simulink library "simetranss"  (R2024b)
settings: Solver=VariableStepAuto  StartTime=0.0  StopTime=10.0  RelTol=1e-3
PostLoadFcn:
  | Ts=1e-6
InitFcn:
  | Ts=1e-6
undefined symbols (not defined in the file): C, C_601, C_603, C_606, CC, Csnu, Csnubber, DiscIntNeverNeededParam, DPL, DPL1ph, FluxTable, ft2km, gcbh, h, Half, Imap2, L, L_601, L_603, L_606, Lbase, LpejoSw, Newton, R_601, R_603, R_606, Raphson, ResistanceM, Roff, Ron, RotorAngles, Rsnu, Rsnubber, Rt4, SampleTime, simetran, sps, sps_rtmsupport, StatorCurrents, T_2wind_ratio, T_Lpu, T_Lpu_pri, T_Rpu, T_Rpu_pri, T_Vpri, T_Vpri_15comp, T_Vsec, Ti, Ts_Power, Z, Zbase, Zm
libraries: fl_lib x248, ee_lib x146, nesl_utility x122, $bdroot x29, simulink x15, eeGeneralControl x2, spsStairGeneratorLib x2, artemis x1
(part 2 of 12)

== system simetranss/Machines ==
  note: Alternative PMSM/BLDC models
  MATE 6/4 SRM : Subsystem  mask(MATE 6/4 Switched Reluctance Motor){MachineType=6/4, Rs=0.05, Inertia=0.05, FluxTable=FluxTable, RotorAngles=RotorAngles, StatorCurrents=StatorCurrents, Friction=0.02, Initialangle=0, TsBlock=-1, nb_points=[100,20,20], PlotCurves=on}
      mask prompts: MachineType "Type:"; Rs "Stator resistance (Ohms):"; Inertia "Inertia (kg.m.m):"; FluxTable "Magnetization characteristic table:"; RotorAngles "Rotor angle vector (degrees):"; StatorCurrents "Stator current vector (A):"; Friction "Friction (N.m.s):"; Initialangle "Initial position (Deg):"; TsBlock "Sample time (-1 for inherited):"; nb_points "Tables Resampling: [flux, angles, currents]"; PlotCurves "Plot magnetization curves"
      mask help:
      | Models a 6/4 switch reluctance motor in MATE-SimScape.
      |
      | See MATE_SwitchedReluctanceMotor64Drive.slx for detailed explanations.
      mask init:
      | block = gcb ;
      | 
      | 
      | %icon
      | x=[-40 -38 -36 -35:5:35  36 38 40];
      | y=round(sqrt(40*40-x.*x));
      | ym=-y;
      | x1=[-35 -33 -31 -30:5:30 31 33 35]/5;
      | y1=round(sqrt(35*35/25-x1.*x1));
      | ym1=-y1;
      | 
      | typ=get_param(block,'MachineType');
      | 
      | table_mode=1;
      | fluxmatfile=FluxTable;
      | srmtype='6/4';
      | theta=RotorAngles;
      | Icoil=StatorCurrents ;
      | currentmap=1;curthetaaxis=1;curfluxaxis=1;torquemap=1;tethetaaxis=1;tecuraxis=1;
      | plotdata=get_param(block,'PlotCurves');
      | init_rotor_pos=[0 -30 -60]+Initialangle;
      | 
      | 
      | [Icoil2,theta2,Imap2, Temap, all_flux_value]=MATE_SRMparam(table_mode,...
      |     fluxmatfile,theta,Icoil,...
      |     currentmap,curthetaaxis,curfluxaxis,...
      |     torquemap,tethetaaxis,tecuraxis,...
      |     srmtype,plotdata,nb_points);
      mask TypeOptions MachineType: 6/4
      mask DialogControl Container2 Prompt: Parameters
  MATE Brushless DC Motor (ALT1) : Subsystem  mask(Round-Rotor PMSM  (Fixed Admittance)){Rs=0.12, Ld=0.003, Mf=0.25366, pp=3, AngInit=0, Ts=Ts}
      mask prompts: Rs "Stator resistance (Ohms)"; Ld "Stator inductance (H)"; Mf "Magnet flux (Wb)"; pp "Number of pairs of poles"; AngInit "Initial mechanical angle (deg)"; Ts "Sample Time (s)"
      mask help:
      | Implements a three-phase round-rotor permanent magnet synchronous machine with stator windings connected in wye to an internal neutral point.
      |
      | Magnet flux is aligned with the d-axis and therefore a sinusoidal back EMF waveform is assumed by the model.
      |
      | The round rotor assumption is equivalent to Ld=Lq. The phase domain inductance matrix is constant in time.
      |
      | This PMSM model is designed with a fixed admittance from the point of view of the SimScape solver and therefore excellent for real-time simulation and HDL coder.
      |
      |
      | Simulink input: Mechanical rotor speed (rad/s)
      |
      | Parameters:
      | Stator resistance in Ohms
      | Stator inductance in Henry (assume Ld=Lq)
      | Magnet flux in Weber: this is the peak magnet flux seen by the stator windings.
      | Number of pairs of poles.
      | Initial angle of the rotor in degrees.
      | Sample time in seconds
  MATE Induction Machine : Subsystem  mask(MATE Induction Machine){Rs=0.5968, Lls=0.0003495, Rr=0.6258, Llr=0.005473, Lm=0.0354, pp=2, Ts=Ts, disc=Backward Euler, park=Stationary, Parameter11=}
      mask prompts: Rs "Stator resistance (Ohms)"; Lls "Stator leakeage inductance (H)"; Rr "Rotor resistance (seen from stator) (Ohms)"; Llr "Rotor leakeage inductance (seen from stator) (H)"; Lm "Mutual inductance (H)"; pp "Number of pairs of poles"; Ts "Sample Time (s)"; disc "Discretization"; park "D-Q reference frame"
      mask help:
      | The MATE induction machine implements a three-phase asynchronous machine (squirrel cage) modeled with a fixed or rotot-based dq reference frame. Stator and rotor windings are connected in wye to an internal neutral point.
      |
      | This model provides a constant admittance to the DAE SimScape solver and make it directly usable in HDL Coder.
      |
      | In particular, there is no matrix inversion occuring in the model when selecting the Stationary frame of reference.
      |
      | Inputs: w_mec: the mechanical frequency of the rotor in rad/s.
      mask init:
      | dis=get_param(gcb,'disc');
      | if isequal(dis,'Backward Euler')
      |     be='on';
      |     ben=1;
      | else
      |     be='off';
      |     ben=0;
      | end
      | 
      | parkk=get_param(gcb,'park');
      | 
      | if isequal(parkk,'Stationary')
      |     park_num=1;
      | else
      |     park_num=0;
      | end
      | 
      | 
      | Lr=Lm+Llr;
      | Ls=Lm+Lls;
      | 
      | invLmat=1/(Lr*Ls-Lm*Lm)*[Lr 0 -Lm 0; 0 Lr 0 -Lm; -Lm 0  Ls  0;  0  -Lm  0  Ls];
      | moinsRmat=-[Rs 0 0 0; 0 Rs 0 0; 0 0  Rr  0;  0  0  0  Rr];
      | Ac=moinsRmat*invLmat;
      | 
      | 
      | 
      | T=[1 0;0 1]*sqrt(2/3)*[1 -0.5 -0.5;0 sqrt(3)/2 -sqrt(3)/2];
      | 
      | T=cat(1,T,[0 0 0; 0 0 0]);
      | 
      | if isequal(be,'off')
      |     Ad=inv(eye(4)-Ts/2*Ac)*(eye(4)+Ts/2*Ac);
      |     Bd=Ts/2*inv(eye(4)-Ts/2*Ac)*T; %trapeze
      |     Bdspeed=inv(eye(4)-Ts/2*Ac)*Ts;
      | else
      |     Ad=inv(eye(4)-Ts*Ac);
      |     Bd=Ts*inv(eye(4)-Ts*Ac)*T;   % euler
      |     Bdspeed=inv(eye(4)-Ts*Ac)*Ts;
      | end
      | 
      | Cd=T'*invLmat;
      | 
      | 
      | Y=Cd*Bd;
      | 
      | % setting external resistances 
      | ResistanceM=zeros(3,3);
      | 
      | Ytot=Y;
      | Yav=(-1/Ytot(1,2)-1/Ytot(1,3)-1/Ytot(2,3))/3;
      | 
      | 
      | ResistanceM(1,2)=Yav;
      | ResistanceM(1,3)=Yav;
      | ResistanceM(2,3)=Yav;
      | 
      | ResistanceM(1,1)=1e12;
      | ResistanceM(2,2)=1e12;
      | ResistanceM(3,3)=1e12;
      mask TypeOptions disc: Backward Euler | Trapezoidal
      mask TypeOptions park: Stationary | Rotor
      mask DialogControl ParameterTabVar0 Prompt: Parameters
      mask DialogControl ParameterTabVar01 Prompt: Advanced parameters
      mask DialogControl Container7 Prompt: More Info
  MATE Permanent Magnet Machine (ALT1) : Subsystem  mask(Permanent Magnet Synchronous Machines (Fixed Admittance)){Rs=0.12, Ld=0.002984, Lq=0.004576, Mf=0.25366, pp=3, AngInit=0, Ts=Ts}
      mask prompts: Rs "Stator resistance (Ohms)"; Ld "Ld d-axis inductance (H)"; Lq "Lq q-axis inductance (H)"; Mf "Magnet flux (Wb)"; pp "Number of pairs of poles"; AngInit "Initial mechanical angle (deg)"; Ts "Sample Time (s)"
      mask help:
      | Implements a three-phase permanent magnet synchronous machine with stator windings connected in wye to an internal neutral point. Magnet flux is aligned with the d-axis and a sinusoidal back EMF waveform is assumed by the model.
      |
      | This PMSM model is designed with a fixed admittance from the point of view of the SimScape solver and therefore excellent for real-time simulation and HDL coder.
      |
      |
      | Simulink input: Mechanical rotor speed (rad/s)
      |
      | Parameters:
      | Stator resistance in Ohms
      | D-axis inductance in Henry
      | Q-axis inductance in Henry
      | Magnet flux in Weber: this is the peak magnet flux seen by the stator windings.
      | Number of pairs of poles.
      | Initial angle of the rotor in degrees.
      | Sample time in seconds
      mask init:
      | cam='on';   % constant admittance  ON
      | ddst='on';  % delayed speed term ON
      | 
      | 
      | invLmat=[1/((Ld+Lq)/2) 0; 0 1/((Ld+Lq)/2) ];
      | moinsRmat=-[Rs 0 ; 0 Rs ];
      | 
      | 
      | T=[1 0;0 1]*sqrt(2/3)*[1 -0.5 -0.5;0 sqrt(3)/2 -sqrt(3)/2];
      | 
      | 
      | if 1==1 %isequal(be,'off')
      |     Bd=Ts/2*inv(eye(2)-Ts/2*moinsRmat*invLmat)*T;%trapeze
      | else
      |     Bd=Ts*inv(eye(2)-Ts*moinsRmat*invLmat)*T;   % euler
      | end
      | 
      | Cd=T'*invLmat;
      | 
      | 
      | Y=Cd*Bd;
      | 
      | % setting external resistances 
      | ResistanceM=zeros(3,3);
      | Ytot=Y; %+Y0;
      | ResistanceM(1,1)= 1/sum(Ytot(1,:));
      | ResistanceM(2,2)= 1/sum(Ytot(2,:));
      | ResistanceM(3,3)= 1/sum(Ytot(3,:));
      | ResistanceM(1,2)=-1/(Ytot(1,2));
      | ResistanceM(1,3)=-1/(Ytot(1,3));
      | ResistanceM(2,1)=-1/(Ytot(2,1));
      | ResistanceM(2,3)=-1/(Ytot(2,3));
      | ResistanceM(3,1)=-1/(Ytot(3,1));
      | ResistanceM(3,2)=-1/(Ytot(3,2));
      | 
      | Lavg=[1/((Ld+Lq)/2) 0; 0 1/((Ld+Lq)/2) ];
      | Rsmat=[-Rs 0 ; 0 -Rs];
      | Adq=Rsmat*Lavg;
      | I=[1 0; 0 1];
      | 
      | Aden=inv(I-Ts/2*Adq);
      | Ad=Aden*(I+Ts/2*Adq);
      | 
      | invLdqDiff=[1/Ld 0; 0 1/Lq]-[1/((Ld+Lq)/2) 0; 0 1/((Ld+Lq)/2) ];
      | RsinvLdqDiff=[-Rs 0 ; 0 -Rs]*invLdqDiff;
  MATE Permanent Magnet Synchronous Machine : Subsystem  mask(Permanent Magnet Synchronous Machines (Fixed Mutual inductance)){Rs=0.12, rtyp=Salient (Ld != Lq), Ld=0.002984, Lq=0.004576, Ldd=0.003, Mf=0.25366, pp=3, AngInit=0, sal_der=0.1, Ts=Ts}
      mask prompts: Rs "Stator resistance (Ohms)"; rtyp "Rotor Type"; Ld "Ld d-axis inductance (H)"; Lq "Lq q-axis inductance (H)"; Ldd "Armature inductance (H)"; Mf "Magnet flux (Wb)"; pp "Number of pairs of poles"; AngInit "Initial mechanical angle (deg)"; sal_der "Saliency derivative time constant (s)"; Ts "Sample Time (s)"
      mask help:
      | Implements a three-phase permanent magnet synchronous machine with stator windings connected in wye to an internal neutral point. Magnet flux is aligned with the d-axis and a sinusoidal back EMF waveform is assumed by the model.
      |
      | This model is implemented as a constant SimScape mutual inductance Lavg=(Ld+Lq)/2 and back-EMF. When Ld is not equal to Lq, the back-EMF part of the flux linkage corresponding to Lq-Ld is computed by the derivative of [(Lq-Ld)/2 0; 0 (Lq-Ld)/2] *Idq with a delay.
      |
      | The 'Saliency derivative time constant' parameter is there to insure the stability of the model relatively to the derivative of the saliency terms. Note that this technique is used in EMTP. See EMTP Theory Book, Synchronous machine section, for more explanations.
      |
      | This PMSM model is designed with a fixed mutual inductance from the point of view of the SimScape solver and therefore excellent for real-time simulation and HDL coder.
      |
      |
      | Simulink input: Mechanical rotor speed (rad/s)
      |
      | Parameters:
      | Stator resistance in Ohms
      | D-axis inductance in Henry
      | Q-axis inductance in Henry
      | Magnet flux in Weber: this is the peak magnet flux seen by the stator windings.
      | Number of pairs of poles.
      | Initial angle of the rotor in degrees.
      | Sample time in seconds
      mask init:
      | block=gcb;
      | visib=get_param(block,'MaskVisibilities');
      | 
      | if isequal (get_param(block,'rtyp'),'Salient (Ld != Lq)')
      |     visib{3}='on';visib{4}='on';visib{5}='off';visib{9}='on';
      | else
      |     visib{3}='off';visib{4}='off';visib{5}='on';visib{9}='off';
      |     Lq=Ldd;
      |     Ld=Ldd;
      |     sal_der=1;
      | end
      | set_param(block,'MaskVisibilities',visib);
      mask Help: eval('open MATE_PMSM_Equations.pdf;');
      mask TypeOptions rtyp: Salient (Ld != Lq) | Round (Ld == Lq)
  MATE Synchronous Machine : Subsystem  mask(MATE Synchronous Machine (Fixed Admittance)){NominalParameters=[ 202e6  13800   60   955 ], Rtype=Salient (5ft order model), Stator=[ 2.9069E-03  3.0892E-04  3.2164E-03 9.7153E-04 0.0], Field=[ 5.9013E-04*0.128/0.08381   3.0712E-04], Dampers1=[ 1.1900E-02  4.9076E-04   2.0081E-02  1.0365E-03  2.0081E-02  1.0365E-03], PolePairs=20, InitialConditions=-95, InitCurrents=[ 1180 9560 9560 9650 [0 -120 120]-95], Ts=Ts, Parameter19=|, sat=off, DiffSat=off, SatVt=[0 0.7 1 1.4], SatIfd=[0 0.5 1 2], plotsat=off, R0=500, X0=0.11643, nsnf_readonly=0.083912, Parameter18=|}
      mask Parameter19=|
      | Saturation: Saturation is used if selected
      |
      | Open stator saturation curve: field current data in per unit of nominal field current
      | Open stator saturation curve: phase-phase RMS terminal voltage in per unit of nominal voltage
      | Plot saturation curves
      | Zero sequence machine reactance (Ohms): grounding impedance internally connected to the stator Y neutral.
      | Neutral grounding resistance (Ohms): grounding resistance (in series with the impedance) internally connected to the stator Y neutral.
      mask Parameter18=|
      | The stator-to-field coil winding turn ratio (Ns_to_Nf) is found using the following formula:
      |
      | Ns_on_Nf=Lmd*I_fn*(2*pi*f_base)/Vbase
      | where Lmd (d-axis mutual inductance), I_fn (nominal field current), f_base (nominal electric frequency) and Vbase (open-stator machine nominal line-line RMS voltage).
      mask prompts: NominalParameters "Nominal power, voltage, frequency, field current  [ Pn(VA) Vn(Vrms) fn(Hz) ifn(A) ]:"; Rtype "Rotor type"; Stator "Stator  [ Rs(ohm), Ll, Lmd, Lmq(H), Lcanay(H) ]:"; Field "Field  [ Rf'(ohm)  Llfd'(H) ]:"; Dampers1 "Dampers   [ Rkd',Llkd'  Rkq1',Llkq1'  Rkq2' Llkq2' ] (R=ohm,L=H): (Rk2 Lfk2 values not used for salient type machine)"; PolePairs "Pole pairs:"; InitialConditions "Initial rotor angle (deg):"; InitCurrents "Initial currents  Ifd (A) Ia Ib Ic (A) (amplitude)  Ia Ib Ic (deg)(angle )"; Ts "Sample Time (s)"; Parameter19 "text1"; sat "Saturation"; DiffSat "Differential saturation (not available)"; SatVt "Open stator saturation curve: phase-phase RMS voltage (pu of nominal voltage)"; SatIfd "Open stator saturation curve: field current (pu of nominal field current)"; plotsat "Plot saturation curves"; R0 "Neutral grounding resistance (Ohms)"; X0 "Zero sequence machine reactance (Ohms)"; nsnf_readonly "Computed Stator/Field turn ratio (read-only)"; Parameter18 "text2"
      mask help:
      | Implements a 3-phase synchronous machine modelled in the dq rotor reference frame for use with SimScape
      | The model uses a fixed admittance matrix method and is well designed for real-time simulation.
      |
      | The model is 6th order for the round rotor type and 5th order for the salient rotor type (Rk2 Llk2 are internally set to inf in this case).Stator windings are connected in wye to an internal neutral point to which an internal impedance to ground can be selected by the user.
      | If selected, saturation occured in both d- and q- axis, using total flux, for the round and salient rotor type.
      |
      |
      | Parameters: (all values are in SI units)
      |
      | Nominal power, voltage, frequency, field current  [ Pn(VA) Vn(Vrms) fn(Hz) ifn(A) ]: nominal values for total power, line-line RMS voltage, frequency and field current
      | Rotor type: Salient (5ft order model)/Round (6th order model)
      | Stator  [ Rs(ohm), Ll, Lmd, Lmq(H) Lcanay(H)]: Stator resistance and leakage inductance, magnetization inductance for d-q axes.The 5th element is the Canay inductance, which can set to 0 if unknown. The Canay inductance applies a correction for the coupling between damper and field windgins in the d-axis.
      | Field  [ Rf'(ohm)  Llfd'(H) ]: Field resistance and leakage inductance (seen from the stator)
      | Dampers   [ Rkd',Llkd'  Rkq1',Llkq1'  Rkq2' Llkq2' ] (R=ohm,L=H): (Rk2 Lfk2 values not used for salient type machine):
      | Pole pairs: number of pair of poles
      | Initial rotor angle  (deg): initial rotor angle in degree.
      | Initial currents  Ifd Ia Ib Ic (A) (amplitude)  Ia Ib Ic (deg)(angle )
      | Sample Time (s) : Sample time of the model in seconds
      mask init:
      | block = gcb;
      | ddst='on';  % delay speed term always in Fixed Admittance model
      | 
      | 
      | 
      | Lmd=Stator(3);
      | Lmq=Stator(4);
      | Lls=Stator(2);
      | Lcanay=0;
      | if length(Stator)==5
      |     Lcanay=Stator(5);
      | end
      |     
      | Ld=Lmd+Lls;
      | Lq=Lmq+Lls;
      | Rs=Stator(1);
      | Rf=Field(1);
      | Llf=Field(2);
      | Lf=Lmd+Llf;
      | Rkd=Dampers1(1);
      | Llkd=Dampers1(2);
      | Lkd=Lmd+Llkd;
      | Rkq=Dampers1(3);
      | Llkq=Dampers1(4);
      | Lkq=Lmq+Llkq;
      | Rkq2=Dampers1(5);
      | Llkq2=Dampers1(6);
      | Lkq2=Lmq+Llkq2;
      | 
      | 
      | 
      | 
      | Lad =1/(1/Lmd+1/Lls+1/Llkd+1/Llf);
      | Laq =1/(1/Lmq+1/Lls+1/Llkq+1/Llkq2);
      | 
      | pp=PolePairs;
      | Sbase=NominalParameters(1);
      | Vbase=NominalParameters(2); % *sqrt(2/3);
      | wbase=NominalParameters(3)*2*pi;
      | Zbase=Vbase*Vbase/Sbase;
      | Ibase=Vbase/Zbase;
      | Lbase=Zbase/wbase;
      | %PhiBase=Lbase*Ibase;
      | PhiBase=Vbase*sqrt(2/3)/wbase;  % real flux base. ref: Gilbert Sybille IREQ
      | I_field_nominal=NominalParameters(4);
      | Ifd_base=I_field_nominal*Lmd/Lbase;
      | 
      | Ns_on_Nf_noLmd=I_field_nominal*wbase/Vbase;
      | Ns_on_Nf=Lmd*I_field_nominal*wbase/Vbase;  % stator/field turn ratio
      | set_param(block,'nsnf_readonly',num2str(Ns_on_Nf));
      | 
      | theta_0=(InitialConditions(1)-90)/180*pi;  % orthonormal Park transform has a 90 deg shift with the conventional SPS Park transform
      | 
      | S=[cos(theta_0) sin(theta_0);-sin(theta_0) cos(theta_0)];
      | 
      | T=S*sqrt(2/3)*[1 -0.5 -0.5;0 sqrt(3)/2 -sqrt(3)/2];
      | 
      | 
      | 
      | % Conversion of initial current phasors to instantaneous values
      | [iau,iao] = pol2cart((InitCurrents(5))*pi/180,InitCurrents(2));
      | [ibu,ibo] = pol2cart((InitCurrents(6))*pi/180,InitCurrents(3));
      | [icu,ico] = pol2cart((InitCurrents(7))*pi/180,InitCurrents(4));
      | 
      | idq=T*(-1)*[iao;ibo;ico];  %-1 here, don't know why exactly...
      | 
      | 
      | 
      | if isequal(get_param(block, 'Rtype'),'Salient (5ft order model)')
      |     nb_row=5;
      |     nb_row3=2;
      |     list_row=[2 5];
      |     Rkq2=0;
      |     Llkq2=inf;
      |     Lkq2=inf;
      |     L0=[Ld 0 Lmd Lmd 0 ; 0 Lq 0 0  Lmq ; Lmd 0 Lf Lmd 0 ; Lmd 0 Lmd Lkd 0  ; 0 Lmq 0 0 Lkq ];
      |     flux_0=L0*[idq;InitCurrents(1)/Ns_on_Nf;0;0]; % initial conditions
      |     dsatOnly=1;  % d-axis saturation only
      |  
      | 
      | MD=(Lmd+Lmq)/2;
      | LD=MD+Lls;
      | LQ=LD;
      | RD=Rs*eye(3);
      | 
      | LDD=[LD MD MD;MD LD MD;MD MD LD];
      | LQQ=[LD MD ;MD LD]; 
      | invD=inv(LDD);
      | RinvD=RD*invD;
      | invQ=[invD(1,1) invD(2,1); invD(2,1) invD(1,1)];
      | 
      | 
      | Yd=invD*inv(eye(3)+Ts/2*RD*invD);
      | Yd22=[Yd(1,1) Yd(1,2); Yd(2,1) Yd(2,2)];
      | 
      | RQ2=2/Ts*inv(Yd22)*(invQ-Yd22)*inv(invQ);
      | 
      | Yq=invQ*inv(eye(2)+Ts/2*RQ2*invQ);
      | 
      | LDx=invD(1,1);
      | MDx=invD(2,1);
      | 
      | RQ=RQ2;
      | 
      | invLavg=[LDx 0 MDx MDx 0; 0 LDx 0 0 MDx ;MDx 0 LDx MDx 0 ;MDx 0 MDx LDx 0 ;0 MDx 0 0 LDx];
      | 
      | Ravg=[Rs 0 0 0 0; 0 RQ(1,1) 0 0 RQ(1,2) ;0 0 Rs 0 0 ;0 0 0 Rs 0 ;0 RQ(1,2) 0 0 RQ(1,1)];
      | RinvLavg=Ravg*invLavg;
      | aaa=RD*invD;
      | bbb=RQ*invQ;
      | RLDx=aaa(1,1);RMDx=aaa(2,1);
      | RLQx=bbb(1,1);RMQx=bbb(2,1);
      | RinvLavg=[RLDx 0 RMDx RMDx 0; 0 RLQx 0 0 RMQx ;RMDx 0 RLDx RMDx 0 ;RMDx 0 RMDx RLDx 0 ;0 RMQx 0 0 RLQx];
      | 
      | 
      | Lmat=[Ld 0 Lmd Lmd 0 ; 0 Lq 0 0  Lmq ; Lmd 0 Lf+Lcanay Lmd+Lcanay 0 ; Lmd 0 Lmd+Lcanay Lkd+Lcanay 0  ; 0 Lmq 0 0 Lkq ];
      | invLmat=inv(Lmat);
      | Rmat=[Rs 0 0 0 0 ; 0 Rs 0 0 0 ; 0 0 Rf  0 0 ; 0 0 0 Rkd 0 ; 0 0 0 0  Rkq ];
      | moinsRmatinvLmat=-Rmat*invLmat;
      | 
      | Ydq=[Yd(1,1) 0 Yd(1,2) Yd(1,3) 0; 0 Yq(1,1) 0 0 Yq(1,2); Yd(2,1) 0 Yd(2,2) Yd(2,3) 0; Yd(3,1) 0 Yd(3,2) Yd(3,3) 0; 0 Yq(2,1) 0 0 Yq(2,2)];
      | 
      | %refine T for the rest...
      | T=[1 0;0 1]*sqrt(2/3)*[1 -0.5 -0.5;0 sqrt(3)/2 -sqrt(3)/2];
      | T=cat(2,T,[0 0]');
      | T=cat(1,T,[0 0 0 1; 0 0 0 0;0 0 0 0]);
      | 
      | 
      | Y44=Ts/2*T'*Ydq*T;
      | Y=Y44(1:3,1:3);
      | 
      | 
      | else
      |     nb_row=6;
      |     nb_row3=3;
      |     list_row=[2 5 6];
      |     L0=[Ld 0 Lmd Lmd 0 0; 0 Lq 0 0  Lmq Lmq; Lmd 0 Lf Lmd 0 0; Lmd 0 Lmd Lkd 0 0 ; 0 Lmq 0 0 Lkq Lmq;0 Lmq 0 0 Lmq Lkq2];
      |     flux_0=L0*[idq;InitCurrents(1)/Ns_on_Nf;0;0;0]; % initial conditions
      |     dsatOnly=0;
      |     Ldq2=(Ld+Lq+Lf+Lkd+Lkq+Lkq2)/6;
      |     Ravg=(Rs+Rs+Rf+Rkd+Rkq+Rkq2)/6;
      |     Lmdq2=(1*Lmd+1*Lmq)/2;
      |     Lavg=[Ldq2 0 Lmdq2 Lmdq2 0 0; 0 Ldq2 0 0 Lmdq2 Lmdq2;Lmdq2 0 Ldq2 Lmdq2 0 0;Lmdq2 0 Lmdq2 Ldq2 0 0;0 Lmdq2 0 0 Ldq2 Lmdq2; 0 Lmdq2 0 0 Lmdq2 Ldq2];
      |     invLavg=inv(Lavg);
      |     
      |     RinvLavg=Ravg*invLavg;
      | Lmat=[Ld 0 Lmd Lmd 0 0; 0 Lq 0 0  Lmq Lmq; Lmd 0 Lf+Lcanay Lmd+Lcanay 0 0; Lmd 0 Lmd+Lcanay Lkd+Lcanay 0 0 ; 0 Lmq 0 0 Lkq Lmq;0 Lmq 0 0 Lmq Lkq2];
      | Rmat=[Rs 0 0 0 0 0; 0 Rs 0 0 0 0; 0 0 Rf  0 0 0; 0 0 0 Rkd 0 0; 0 0 0 0  Rkq 0; 0 0 0 0 0 Rkq2];
      | invLmat=inv(Lmat);
      | moinsRmatinvLmat=-Rmat*invLmat;
      | 
      | % Yd=invD*inv(eye(3)+Ts/2*RD*invD);
      | % Yd22=[Yd(1,1) Yd(1,2); Yd(2,1) Yd(2,2)];
      | % 
      | % RQ2=2/Ts*inv(Yd22)*(invQ-Yd22)*inv(invQ);
      | % 
      | % Yq=invQ*inv(eye(2)+Ts/2*RQ2*invQ);
      | 
      | %refine T for the rest... one more row of 0 here...
      | T=[1 0;0 1]*sqrt(2/3)*[1 -0.5 -0.5;0 sqrt(3)/2 -sqrt(3)/2];
      | T=cat(2,T,[0 0]');
      | T=cat(1,T,[0 0 0 1; 0 0 0 0;0 0 0 0; 0 0 0 0]);
      | 
      | %Ts/2*Ravg*invLavg
      | Ydq=invLavg*inv(eye(6)+Ts/2*Ravg*invLavg);
      | Y44=Ts/2*T'*Ydq*T;
      | Y=Y44(1:3,1:3);
      | 
      | 
      | end
      | 
      | % zero-sequence admittance
      | T0=[1 1 1]*sqrt(1/3);
      | invL0=wbase/X0;
      | Ac0=-(Rs+R0)*invL0;
      | Y0=Ts/2*T0'*invL0*inv(1-Ts/2*Ac0)*T0;
      | 
      | % setting external resistances 
      | ResistanceM=zeros(3,3);
      | Ytot=Y+Y0;
      | ResistanceM(1,1)= 1/sum(Ytot(1,:));
      | ResistanceM(2,2)= 1/sum(Ytot(2,:));
      | ResistanceM(3,3)= 1/sum(Ytot(3,:));
      | ResistanceM(1,2)=-1/(Ytot(1,2));
      | ResistanceM(1,3)=-1/(Ytot(1,3));
      | ResistanceM(2,1)=-1/(Ytot(2,1));
      | ResistanceM(2,3)=-1/(Ytot(2,3));
      | ResistanceM(3,1)=-1/(Ytot(3,1));
      | ResistanceM(3,2)=-1/(Ytot(3,2));
      | 
      | 
      | 
      | 
      | 
      | Ifd=str2num(get_param(block,'SatIfd'));
      | Vt=str2num(get_param(block,'SatVt'));
      | Ifd=Ifd*I_field_nominal;   % modif 17 mai 2017: Vt=f(Ifd) en pu
      | Vt=Vt*Vbase;
      | if sat==0
      |     set_param(block,'DiffSat','off');
      | end
      | 
      | if sat==1
      |     %Vbase=NominalParameters(2);
      |     %wbase=NominalParameters(3)*2*pi;
      |     %PhiBase=Vbase*sqrt(2/3)/wbase;  % real flux base ref: Gilbert Sybille IREQ
      |     %I_field_nominal=NominalParameters(4);
      |     %Ns_on_Nf=Lmd*I_field_nominal*wbase/Vbase;  % stator/field turn
      |     
      |     if length(Ifd)~=length(Vt)
      |         error('Saturation field current and voltage must have the same length');
      |     end
      |     if length(Ifd)<2
      |         error('Saturation field current and voltage must have a minimum length of 2, including the (0,0) point');
      |     end
      |     if Ifd(1)~=0 | Vt(1)~=0
      |         error('Saturation field current and voltage must include the (0,0) point');
      |     end
      |     
      |     %Vt=Lmd*I_field_nominal*wbase/Ns_on_Nf;
      |     %Lmd_sat=Vt*Ns_on_Nf/Ifd/wbase;
      |     % find nominal magnetizing inductance from the saturation curve
      |     for i=2:length(Ifd)
      |         if Ifd(i)>I_field_nominal
      |             break
      |         end
      |     end
      |     pente=(Vt(i)-Vt(i-1))/(Ifd(i)-Ifd(i-1));
      |     Vtnom_sat=Vt(i-1)+(I_field_nominal-Ifd(i-1))*pente;
      |     Lnom=Vtnom_sat/I_field_nominal;  % slope at nominal field current
      |     table_saturation_factor=(Vt(2:end)./Ifd(2:end))/Lnom;
      |     table_saturation_factor=[table_saturation_factor(1) table_saturation_factor];
      |     % careful with point 0,0...
      |     %table_flux_input=Vt*sqrt(2/3)/wbase;
      |     table_flux_input=Vt/wbase;  % the sqrt(2/3) factor is not required here
      |     
      | else
      |     table_saturation_factor=[1 1 1];
      |     table_flux_input=[0 1 2];
      |     
      | end
      | 
      | Vx=Vt'/wbase;
      | b=Ifd'/Ns_on_Nf;
      | 
      | if DiffSat==1
      |     if length(Ifd)~=4
      |         error('When using differential saturation, saturation field current and voltage must be a vector of 4 of length');
      |     end
      |     
      |     
      |     %Lmd=(Vf/wbase)/(Ifd/Ns_on_Nf)
      | 
      |     
      |     A(:,1)=[1 1 1 1]';
      |     A(:,2)=Vx';
      |     A(:,3)=(Vx.*Vx)';
      |     A(:,4)=(Vx.*Vx.*Vx)';
      |     
      |     w=inv(A)*b;
      | else
      |     w=[1;1;1;1];
      |     
      | end
      | 
      | 
      | if plotsat
      |     figure
      |     if DiffSat==1
      |         x=0:Vx(end)/20:Vx(end);
      |         y=w(1)+x.*w(2)+x.*x.*w(3)+x.*x.*x.*w(4);  %fitted curve i=f(v) car on veut une fonction de v (ou flux)
      |         plot(b*Ns_on_Nf,Vx*wbase,'*b');
      |         hold on
      |         plot(y*Ns_on_Nf,x*wbase,'r');  % put current on x-axis
      |         xlabel('Field current (A)');
      |         ylabel('Open stator terminal voltage (V)');
      |         
      |         slopee=w(2)+2*w(3).*Vx+3*w(4).*Vx.*Vx;
      |         offsett=w(1)-w(3).*Vx.*Vx-2*w(4).*Vx.*Vx.*Vx;
      |         slope_inv=1./slopee;
      |         offset_inv=-offsett./slopee;  % pente et offset de la courbe v=f(i)
      |         ifdvec=0:b(end)/20:b(end);
      |         for ii=2:length(slope_inv)
      |             vv=offset_inv(ii)+slope_inv(ii).*ifdvec;
      |             plot(ifdvec*Ns_on_Nf,vv*wbase,'g');
      |         end
      |         legend('user data point','fitted curve','linear approx at user points','Location','NorthWest')
      |         
      |         
      |         hold off
      |         
      |     else
      |         plot(b*Ns_on_Nf,Vx*wbase,'*-b');
      |         hold
      |         plot([I_field_nominal I_field_nominal],[0 Vbase],'-r');
      |         plot([0 I_field_nominal],[Vbase Vbase],'-r');
      |         xlabel('Field current (A)');
      |         ylabel('Open stator terminal voltage (V)');
      |         title ('red line indicate nominal point');
      |         hold off
      |     end   
      | end
      |     set_param(block,'plotsat', 'off');
      | 
      | 
      | 
      | % set model speed term routing
      | if isequal(ddst, 'on')
      |     o1=0;
      |     o2=1:(nb_row+4);
      | 
      | else
      |     o1=1;
      |     o2=1:4;
      | 
      | end
      mask TypeOptions Rtype: Salient (5ft order model) | Round (6th order model)
      mask Callback sat:
      | block = gcb;
      | sattt=get_param(block,'sat');
      | 
      | % hide saturation option if saturation not selected
      | visib=get_param(block,'MaskVisibilities');
      | if isequal(sattt,'on')
      |     visib{12}='off';visib{13}='on';visib{14}='on';visib{15}='on';
      | else
      |     visib{12}='off';visib{13}='off';visib{14}='off';visib{15}='off';
      | end
      | visib{11}='on';
      | set_param(block,'MaskVisibilities',visib);
      mask DialogControl ParameterTabVar0 Prompt: Parameters
      mask DialogControl Container5 Prompt: Saturation and zero sequence
      mask DialogControl ParameterTabVar01 Prompt: More Info
  Mechanical model : Subsystem  mask(Machine rotational mechanical model){J=0.016731, F=0, fo=0, Ts=Ts, Parameter5=|}
      mask Parameter5=|
      | Conversion from Per-Unit values
      |
      | J=2*H*Pn/w_mec^2
      | F=D*Pn/w_mec^2
      | where:
      | J is the inertia in km.m^2
      | H is the inertia constant in seconds.
      | F is the friction factor in N.m.s
      | D in the friction factor or damping factor in pu.
      | Pn is the nominal power of the machine
      | w_mec is the nominal mechanical rotational frequency of the machine in rad/s
      mask prompts: J "Inertia (kg.m^2)"; F "Friction (N.m.s)"; fo "Initial mechanical frequency (Hz)"; Ts "Sample Time (s)"
      mask help:
      | This block can implement the mechanical equation of rotating machines.
      |
      | The block working equation is:
      | wmec=1/J*INTEGRAL{( Te - Tm -F*wmec )*dt}
      |
      | Parameters:
      | Inertia J (kg.m^2)
      | Friction F (N.m.s)
      | Initial mechanical frequency (Hz)
      | Sample Time (s).
      |
      | Signals:
      | Te: electric torque input from the machine (N.m.)
      | Tm : mechanical torque applied to the shaft (N.m.)
      | wmec: mechanical speed of machine (rad/s)
      mask DialogControl Container3 Prompt: Per-Unit Help

== system simetranss/Measure ==
  Bus Measure : Subsystem  mask(SimScape Three-Phase VI Measurement){VoltageMeasurement=phase-to-ground, SetLabelV=on, LabelV=Vabc_B1ssc, Vpu=off, VpuLL=off, CurrentMeasurement=yes, SetLabelI=on, LabelI=Iabc_B1ssc, Ipu=off, Pbase=100e6, Vbase=500e3, bnumber=622, dis=off}
      mask prompts: VoltageMeasurement "Voltage measurement"; SetLabelV "Use a label"; LabelV "Signal label  (use a From block to collect this signal)"; Vpu "Voltages in pu,  based on peak value of nominal phase-to-ground voltage"; VpuLL "Voltages in pu,  based on peak value of nominal phase-to-phase  voltage"; CurrentMeasurement "Current measurement"; SetLabelI "Use a label"; LabelI "Signal label  (use a From block to collect this signal)"; Ipu "Currents in pu"; Pbase "Base power ( VA 3 phase)"; Vbase "Nominal voltage used for pu measurement (Vrms phase-phase) :"; bnumber "Bus number"; dis "Disable measurements"
      mask help:
      | Three-phase voltage and current measurements.
      |
      | The block can output the voltages and currents in per unit values or in volts and amperes.
      mask init:
      | mess=['Bus ' bnumber ];
      | %xxx=fprintf('Sum = %d', 7);
      | block = gcb;
      | block2=[block '/Measure'];
      | Kv=1;
      | Ki=1;
      | 
      | [Kv ,Ki ]=MATE3phVIMeasurementParams(block ,Vpu ,VpuLL ,Ipu ,Vbase ,Pbase,block2);
      | MATE3phVIMeasurementCb(block ,block);
      | 
      | 
      | vtype=get_param(block,'VoltageMeasurement');
      | if isequal(vtype,'phase-to-phase')
      |     str='ee.enum.vmeasurement.ll';
      | else
      |     str= 'ee.enum.vmeasurement.lg';
      | end
      | set_param([block2 '/Meas'],'vMeasurementType',str);
      | 
      | type=get_param(block,'dis');
      | if isequal(type,'on')
      |     set_param([block '/Pass'], 'Commented', 'off');
      |     set_param([block '/Measure'], 'Commented', 'on');
      | else
      |     set_param([block '/Pass'], 'Commented', 'on');
      |     set_param([block '/Measure'], 'Commented', 'off');
      | end
      mask TypeOptions VoltageMeasurement: no | phase-to-ground | phase-to-phase
      mask TypeOptions CurrentMeasurement: no | yes
      mask Display:
      | %disp('bus')
      | %disp(block2)
      | fprintf('bus %s', get_param(gcb,'bnumber'));
  Current Mesure : Subsystem  mask(SimScape Current Measurement){SetLabelV=on, LabelV=Ia, bnumber=node2}
      mask prompts: SetLabelV "Use a label"; LabelV "Signal label  (use a From block to collect this signal)"; bnumber "Identifier"
      mask help: A current measurement with Goto-From capability and Simulink output (no PS-Simulink converter needed!)
      mask init:
      | mess=[bnumber];
      | %xxx=fprintf('Sum = %d', 7);
      | block = gcb;
      | v =get_param (block ,'MaskVisibilities' ); 
      | 
      | 
      | 
      | %MATEVIMeasurementCb(block);
      | 
      | WantVlabel =strcmp ('on' ,get_param (block ,'SetLabelV' )); 
      | 
      | 
      | Vabc =get_param ([block ,'/I' ],'Blocktype' ); 
      | 
      | if WantVlabel
      |     v{2}='on';
      |     if ~strcmp (Vabc ,'Goto' )
      |         replace_block (block ,'LookUnderMasks' ,'on' ,'FollowLinks' ,'on' ,'Name' ,'I' ,'goto' ,'noprompt' );
      |     end
      |     set_param ([block ,'/I' ],'GotoTag' ,get_param (block ,'LabelV' ),'TagVisibility' ,'Global' );
      | else
      |     v{2}='off';
      |     if ~strcmp (Vabc ,'Outport' )
      |         replace_block (block ,'LookUnderMasks' ,'on' ,'FollowLinks' ,'on' ,'Name' ,'I' ,'Outport' ,'noprompt' );
      |         set_param ([block ,'/I' ],'Port' ,'1' );
      |     end
      | end
      | 
      | set_param (block ,'MaskVisibilities',v);
      mask Display: fprintf('Current\n %s', get_param(gcb,'bnumber'));
  Voltage Mesure : Subsystem  mask(SimScape Voltage Measurement){SetLabelV=on, LabelV=Va, bnumber=node1}
      mask prompts: SetLabelV "Use a label"; LabelV "Signal label  (use a From block to collect this signal)"; bnumber "Identifier"
      mask help: A voltage measurement with Goto-From capability and Simulink output (no PS-Simulink converter needed!)
      mask init:
      | block = gcb;
      | 
      | 
      | 
      | %MATEVIMeasurementCb(block);
      | 
      | WantVlabel =strcmp ('on' ,get_param (block ,'SetLabelV' )); 
      | v =get_param (block ,'MaskVisibilities' ); 
      | 
      | 
      | Vabc =get_param ([block ,'/V' ],'Blocktype' ); 
      | 
      | if WantVlabel
      |     v{2}='on';
      |     if ~strcmp (Vabc ,'Goto' )
      |         replace_block (block ,'LookUnderMasks' ,'on' ,'FollowLinks' ,'on' ,'Name' ,'V' ,'goto' ,'noprompt' );
      |     end
      |     set_param ([block ,'/V' ],'GotoTag' ,get_param (block ,'LabelV' ),'TagVisibility' ,'Global' );
      | else
      |     v{2}='off';
      |     if ~strcmp (Vabc ,'Outport' )
      |         replace_block (block ,'LookUnderMasks' ,'on' ,'FollowLinks' ,'on' ,'Name' ,'V' ,'Outport' ,'noprompt' );
      |         set_param ([block ,'/V' ],'Port' ,'1' );
      |     end
      | end
      | set_param (block ,'MaskVisibilities',v );
      mask Display: fprintf('Voltage\n %s', get_param(gcb,'bnumber'));
  bus : Subsystem  mask{bn=611}
      mask prompts: bn "Bus number"
      settings: AttributesFormatString=Bus %<bn>
  bus2 : Subsystem  Commented=on  mask(Bus number){bn=646}
      mask prompts: bn "Bus number"
      settings: AttributesFormatString=Bus %<bn>

== system simetranss/Misc ==
  Discrete Mean value : Subsystem  LoadFcn=sps_rtmsupport('LoadFcn', gcbh);  StartFcn=sps_rtmsupport('StartFcn', gcbh);  StopFcn=sps_rtmsupport('StopFcn', gcbh);  mask(Mean){Freq=sps.Freq, Vinit=sps.Real_Init, Ts=Ts}
      mask prompts: Freq "Fundamental frequency (Hz):"; Vinit "Initial input (DC component):"; Ts "Sample time:"
      mask help: Compute the mean value of the input signal over a running window of one cycle of the specified fundamental frequency. For the first cycle of simulation, the output is held constant to the specified initial input value.
      mask init:
      | block=gcb;
      | mate.Freq =Freq ; 
      | mate.Vinit =Vinit ; 
      | 
      | SamplesPerCycle =1 ./Freq /Ts ; 
      | RoundSamplesPerCycle =ceil (SamplesPerCycle ); 
      | mate.Delay =RoundSamplesPerCycle *Ts ; 
      | Corr1 =(SamplesPerCycle -RoundSamplesPerCycle )/2 ; 
      | Corr2 =(SamplesPerCycle -RoundSamplesPerCycle )./SamplesPerCycle ; 
      | mate.K1 =Corr1 .*Corr2 ; 
      | mate.K2 =Corr2 +Corr1 .*Corr2 ;
      settings: CopyFcn=sps_rtmsupport('CopyFcn', gcbh);  DeleteFcn=sps_rtmsupport('DeleteFcn', gcbh);  UndoDeleteFcn=sps_rtmsupport('UndoDeleteFcn', gcbh);  ModelCloseFcn=sps_rtmsupport('ModelCloseFcn', gcbh);  PreSaveFcn=sps_rtmsupport('PreSaveFcn', gcbh);  PostSaveFcn=sps_rtmsupport('PostSaveFcn', gcbh);  NameChangeFcn=sps_rtmsupport('NameChangeFcn', gcbh);  PreCopyFcn=sps_rtmsupport('PreCopyFcn', gcbh);  OpenFcn=sps_rtmsupport('OpenFcn', gcbh, []);  CloseFcn=sps_rtmsupport('CloseFcn', gcbh);  PreDeleteFcn=sps_rtmsupport('PreDeleteFcn', gcbh);
      mask Help: helpview(psbhelp);
      mask Display:
      | plot(0,0, 1,1)
      | plot([0.8 1], [0.75 0.75])
      | plot([0.85 .95], [0.35 0.65],[0.85 .95], [0.65 0.35])
  Fourier : Subsystem  LoadFcn=sps_rtmsupport('LoadFcn', gcbh);  StartFcn=sps_rtmsupport('StartFcn', gcbh);  StopFcn=sps_rtmsupport('StopFcn', gcbh);  mask(Fourier){Freq=sps.Freq, n=1, ParInit=sps.Par_Init_RMS, Ts=Ts}
      mask prompts: Freq "Fundamental frequency (Hz):"; n "Harmonic n (0=DC, 1=fundamental):"; ParInit "Initial input [ Mag, Phase (degrees) ]:"; Ts "Sample time:"
      mask help:
      | Fourier analysis of the input signal over a running window of one cycle of the fundamental frequency.
      |
      | For the first cycle of simulation, the outputs are held  to the value specified in the Initial input parameter.
      mask init:
      | block=gcb;
      | BK =strrep (block ,char (10 ),char (32 )); 
      | 
      | if (Freq <=0 )
      | error('Frequency must be greater than 0') 
      | end
      | if (n <0 )
      | error ('Harmonic number must greater or equal to 0'); 
      | end
      | if size (ParInit ,2 ) ~=2 
      | error ('Initial value mus be a vector of 2'); 
      | end
      | 
      | mate.Freq =Freq ; 
      | mate.n =n ; 
      | mate.k =2 -(n ==0 ); 
      | mate.Real_Init =ParInit (:,1 ).*cos (pi /180 .*ParInit (:,2 )); 
      | mate.Imag_Init =ParInit (:,1 ).*sin (pi /180 .*ParInit (:,2 ));
      settings: CopyFcn=sps_rtmsupport('CopyFcn', gcbh);  DeleteFcn=sps_rtmsupport('DeleteFcn', gcbh);  UndoDeleteFcn=sps_rtmsupport('UndoDeleteFcn', gcbh);  ModelCloseFcn=sps_rtmsupport('ModelCloseFcn', gcbh);  PreSaveFcn=sps_rtmsupport('PreSaveFcn', gcbh);  PostSaveFcn=sps_rtmsupport('PostSaveFcn', gcbh);  NameChangeFcn=sps_rtmsupport('NameChangeFcn', gcbh);  PreCopyFcn=sps_rtmsupport('PreCopyFcn', gcbh);  OpenFcn=sps_rtmsupport('OpenFcn', gcbh, []);  CloseFcn=sps_rtmsupport('CloseFcn', gcbh);  PreDeleteFcn=sps_rtmsupport('PreDeleteFcn', gcbh);
      mask Help: helpview(psbhelp);
      mask Display:
      | port_label('output',1,'|u|')
      | port_label('output',2,'\angleu', 'texmode', 'on')
  RMS : Subsystem  LoadFcn=sps_rtmsupport('LoadFcn', gcbh);  StartFcn=sps_rtmsupport('StartFcn', gcbh);  StopFcn=sps_rtmsupport('StopFcn', gcbh);  mask(RMS){TrueRMS=off, Freq=60, RMSInit=0, Ts=Ts}
      mask prompts: TrueRMS "True RMS value"; Freq "Fundamental frequency (Hz):"; RMSInit "Initial RMS value:"; Ts "Sample time:"
      mask help:
      | Measure the true root mean square (RMS) value of the input signal at the specified fundamental frequency.
      |
      | When True RMS value parameter is unchecked, the block outputs the RMS value of the fundamental component of the input signal.
      mask init:
      | mate.TrueRMS =TrueRMS ; 
      | if TrueRMS ==1 
      | mate.PortName ='TrueRMS' ; 
      | else
      | mate.PortName ='RMS' ; 
      | end
      | 
      | 
      | 
      | 
      | 
      | if (Freq <=0 )
      | error('Frequency must be greater than 0')
      | end
      | 
      | 
      | mate.Freq =Freq ; 
      | 
      | mate.RMSInit_TrueRMS =RMSInit .*RMSInit ; 
      | mate.RMSInit_RMS =cat (2 ,(RMSInit .*sqrt (2 ))' ,zeros (1 ,length (RMSInit ))' );
      settings: CopyFcn=sps_rtmsupport('CopyFcn', gcbh);  DeleteFcn=sps_rtmsupport('DeleteFcn', gcbh);  UndoDeleteFcn=sps_rtmsupport('UndoDeleteFcn', gcbh);  ModelCloseFcn=sps_rtmsupport('ModelCloseFcn', gcbh);  PreSaveFcn=sps_rtmsupport('PreSaveFcn', gcbh);  PostSaveFcn=sps_rtmsupport('PostSaveFcn', gcbh);  NameChangeFcn=sps_rtmsupport('NameChangeFcn', gcbh);  PreCopyFcn=sps_rtmsupport('PreCopyFcn', gcbh);  OpenFcn=sps_rtmsupport('OpenFcn', gcbh, [1]);  CloseFcn=sps_rtmsupport('CloseFcn', gcbh);  PreDeleteFcn=sps_rtmsupport('PreDeleteFcn', gcbh);
      mask Help: helpview(psbhelp);
      mask Display: color('blue');disp('RMS')
